simulink model "ImplementationDiscreteController"  (Simulink 7.3)
settings: Solver=ode45  StartTime=0.0  StopTime=50  FixedStep=Ts  MaxStep=Ts  RelTol=1e-3
PostLoadFcn:
  | , if any(exist('dsrtsu_mdlpostloadfcn', 'file') == [2, 3, 6]), try dsrtsu_mdlpostloadfcn('Execute', bdroot); catch fprintf('Error in PostLoadFcn (dsrtsu_mdlpostloadfcn) for model "%s":\n %s\n', bdroot, lasterr); end, end,
undefined symbols (not defined in the file or in its folder): Cd_den, Cd_num, DiscIntNeverNeededParam, I0, P_den, P_num, Ts, Y0
settings Model: DSRTSU_INTERNAL_RTI_VER=350  DSRTSU_INTERNAL_RTI_TYPE=rti1104  Creator=whendrix  LastModifiedBy=Control  BufferReuse=off
settings OptimizationCC: BlockReduction=off  OptimizeBlockIOStorage=off  BufferReuse=off  ExpressionFolding=off  LocalBlockOutputs=off
settings HardwareCC: ProdIntDivRoundTo=Zero  ProdEndianess=BigEndian  ProdHWDeviceType=Generic->Custom  TargetIntDivRoundTo=Zero  TargetEndianess=BigEndian  TargetHWDeviceType=Generic->Custom
settings RTWCC: SystemTargetFile=rti1104.tlc  MakeCommand=make_rti  TemplateMakefile=rti1104.tmf  Description=dSPACE DS1104 Hardware Platform  ProcessScript=rti1104_make_rtw_hook
settings STFCustomTargetCC: MatFileLogging=on  SystemTargetFile=rti1104.tlc
settings GRTTargetCC: ParMdlRefBuildCompliant=off  CompOptLevelCompliant=off  ExtModeMexFile=noextcomm
settings CustomProperty: DataType=RTWOptions_EnumType_C__dSPACE6p5_matlab_rti1104_tlc_rti1104_1InitialSimState  Value=RUN
settings EnumStrPairs: String=RUN

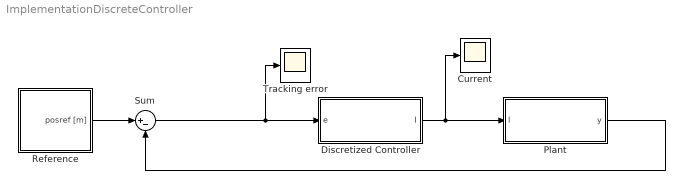
== system ImplementationDiscreteController ==
  Current : Scope
      settings: TimeRange=50
  Discretized Controller : Subsystem
  Plant : Subsystem
  Reference : Subsystem
  Sum : Sum  Inputs=|+-  OutDataType=fixdt(1, 16)  OutScaling=2^0
  Tracking error : Scope
      settings: TimeRange=50
  wires:
  Sum/1 -> Tracking error/1, Discretized Controller/1(e)
  Plant/1(y) -> Sum/2
  Reference/1(posref [m]) -> Sum/1
  Discretized Controller/1(I) -> Plant/1(I), Current/1

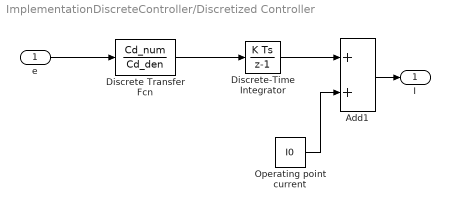
== system ImplementationDiscreteController/Discretized Controller ==
  e : Inport  OutDataType=fixdt(1, 16)  OutScaling=2^0
  Add1 : Sum  OutDataType=fixdt(1, 16)  OutScaling=2^-10
  Discrete Transfer Fcn : DiscreteTransferFcn  Numerator=Cd_num  Denominator=Cd_den  SampleTime=Ts
  Discrete-Time Integrator : DiscreteIntegrator  gainval=1/Ts  SampleTime=Ts  OutDataType=fixdt(1, 16)  OutScaling=2^0  LimitOutput=on  UpperSaturationLimit=3-I0  LowerSaturationLimit=-I0  ICPrevOutput=DiscIntNeverNeededParam  ICPrevScaledInput=DiscIntNeverNeededParam
  Operating point current : Constant  Value=I0  OutDataType=fixdt(1, 16)  OutScaling=2^0
  I : Outport  OutDataType=fixdt(1, 16)  OutScaling=2^0
  wires:
  Operating point current/1 -> Add1/2
  Discrete-Time Integrator/1 -> Add1/1
  Add1/1 -> I/1
  Discrete Transfer Fcn/1 -> Discrete-Time Integrator/1
  e/1 -> Discrete Transfer Fcn/1

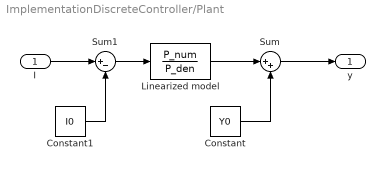
== system ImplementationDiscreteController/Plant ==
  I : Inport  OutDataType=fixdt(1, 16)  OutScaling=2^0
  Constant : Constant  Value=Y0  OutDataType=fixdt(1, 16)  OutScaling=2^0
  Constant1 : Constant  Value=I0  OutDataType=fixdt(1, 16)  OutScaling=2^0
  Linearized model : TransferFcn  Numerator=P_num  Denominator=P_den
  Sum : Sum  Inputs=|++  OutDataType=fixdt(1, 16)  OutScaling=2^0
  Sum1 : Sum  Inputs=|+-  OutDataType=fixdt(1, 16)  OutScaling=2^0
  y : Outport  OutDataType=fixdt(1, 16)  OutScaling=2^0
  wires:
  Linearized model/1 -> Sum/1
  Sum/1 -> y/1
  Constant/1 -> Sum/2
  Sum1/1 -> Linearized model/1
  Constant1/1 -> Sum1/2
  I/1 -> Sum1/1

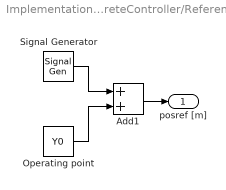
== system ImplementationDiscreteController/Reference ==
  Add1 : Sum  OutDataType=fixdt(1, 16)  OutScaling=2^-10
  Operating point : Constant  Value=Y0  OutDataType=fixdt(1, 16)  OutScaling=2^0
  Signal Generator : SignalGenerator  WaveForm=square  Amplitude=5e-4  Frequency=0.5
  posref [m] : Outport
  wires:
  Signal Generator/1 -> Add1/1
  Add1/1 -> posref [m]/1
  Operating point/1 -> Add1/2
